simulink library "ctc"  (Simulink 8.1)
settings: Solver=ode1  StartTime=0.0  StopTime=Inf  FixedStep=0.001  RelTol=1e-3
PostLoadFcn:
  | , if any(exist('dsrtsu_mdlpostloadfcn', 'file') == [2, 3, 6]), try dsrtsu_mdlpostloadfcn('Execute', bdroot); catch fprintf('Error in PostLoadFcn (dsrtsu_mdlpostloadfcn) for model "%s":\n %s\n', bdroot, lasterr); end, end,
undefined symbols (not defined in the file or in its folder): ENUM_ACCSTATE_STANDSTILL, KACC_BackToTqMinDecel_mps2, ZERO_FLOAT
libraries: ctp x1, trs x1, ptc x1, ltt x1, tpl x1, tru x1, trl x1
settings Model: DSRTSU_INTERNAL_RTI_VER=450  DSRTSU_INTERNAL_RTI_TYPE=rti1401  RTICANMMDATA=struct('GeneralSetupData',struct('modelroot','D:\ELN150201_TAIWAN\trunk\AdasDragon\software\sw_development\arch\app\acc','generalsettings',struct('filesettings',struct('destfolder',struct('Name','RTICANMM_FILES','Check',1),'buildfolder',struct('Name','.','Check',1),'AbsDestfolder',struct('Name','D:\ELN150201_TAIWAN\trunk\AdasDragon\software\sw_development\arch\app\acc\RTICANMM_FILES'),'AbsBuildfolder',struct('Name','D:\ELN150201_TAIWAN\trunk\AdasDragon\software\sw_development\arch\app\acc'))),'options',struct('addpaths',1,'rmpaths',1,'addtrcexclusion',logical(1),'cannavigator',struct('checkmonitoring',0),'show_usrtrc',0,'use_usrtrc',0),'advanced',struct('options',[1 1 1 1 1 1 1 1 1 1 1 1 1 1 1 1 1 1 1 1 1 1 1 1 1 1 1 1 1 1 1 1 1 1 1 1 1 1 1 1 1 1 1 1 1 1 1 1 1 1 1 1 1 1 1 1 1 1 1 1 1 1 1 1 1 1 1 1 1 1 1 1 1 1 1 1 1 1 1 1 1 1 1 1 1 1 1 1 1 1 1 1 1 1 1 1 1 1 1 1]),'MPSetup',{{}},'modelname','ctc','block','ctc'))  DSRTSU_INTERNAL_RTIFPGA=40  Creator=tescamilla  LastModifiedBy=AT015555

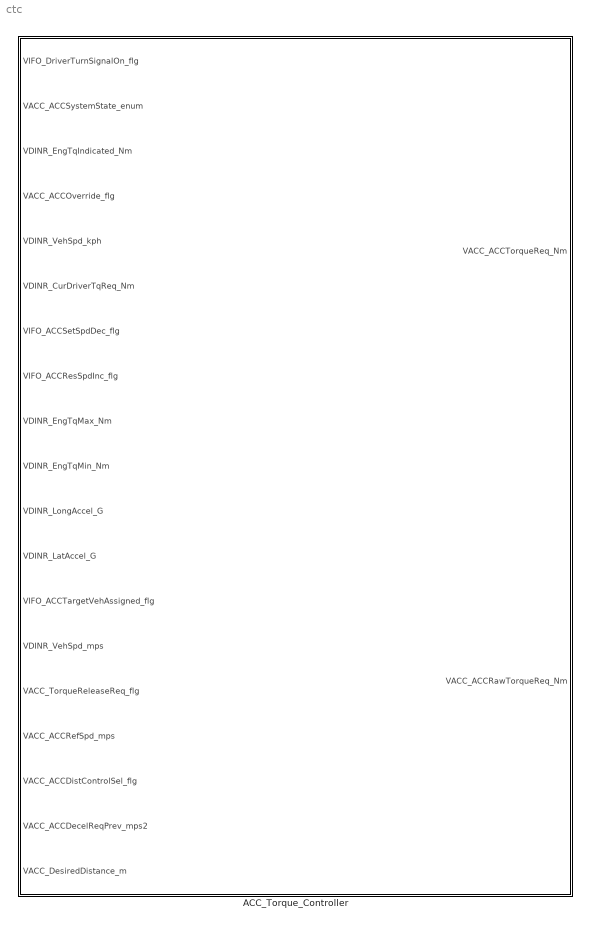
== system ctc ==
  ACC_Torque_Controller : Subsystem

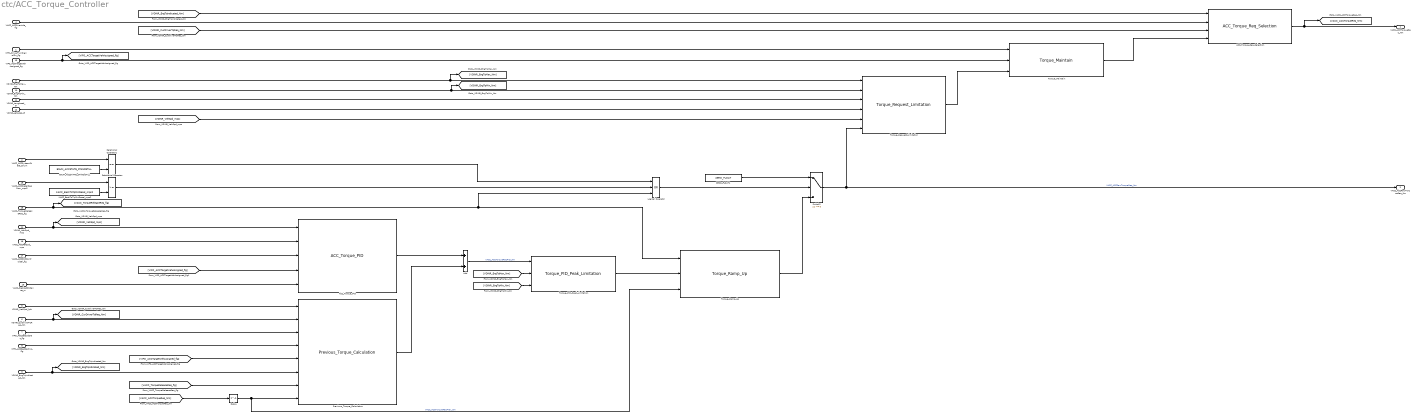
== system ctc/ACC_Torque_Controller ==
  VIFO_DriverTurnSignalOn_flg : Inport
  VACC_ACCSystemState_enum : Inport  Port=2
  VDINR_EngTqIndicated_Nm : Inport  Port=3
  VACC_ACCOverride_flg : Inport  Port=4
  VDINR_VehSpd_kph : Inport  Port=5
  VDINR_CurDriverTqReq_Nm : Inport  Port=6
  VIFO_ACCSetSpdDec_flg : Inport  Port=7
  VIFO_ACCResSpdInc_flg : Inport  Port=8
  VDINR_EngTqMax_Nm : Inport  Port=9
  VDINR_EngTqMin_Nm : Inport  Port=10
  VDINR_LongAccel_G : Inport  Port=11
  VDINR_LatAccel_G : Inport  Port=12
  VIFO_ACCTargetVehAssigned_flg : Inport  Port=13
  VDINR_VehSpd_mps : Inport  Port=14
  VACC_TorqueReleaseReq_flg : Inport  Port=15
  VACC_ACCRefSpd_mps : Inport  Port=16
  VACC_ACCDistControlSel_flg : Inport  Port=17
  VACC_ACCDecelReqPrev_mps2 : Inport  Port=18
  VACC_DesiredDistance_m : Inport  Port=19
  ACC_Torque_PID : ctp/ACC_Torque_PID
  ACC_Torque_Req_Selection : trs/ACC_Torque_Req_Selection
  Add : Sum
  Delay : Delay  DelayLength=1  InitialCondition=0
  ENUM_ACCSTATE_STANDSTILL : Constant  Value=ENUM_ACCSTATE_STANDSTILL
  KACC_BackToTqMinDecel_mps2 : Constant  Value=KACC_BackToTqMinDecel_mps2
  Logical Operator : Logic  Operator=OR  Inputs=3  AllPortsSameDT=off  OutDataTypeStr=boolean
  Previous_Torque_Calculation : ptc/Previous_Torque_Calculation
  Relational Operator : RelationalOperator  OutDataTypeStr=boolean
  Relational Operator1 : RelationalOperator  Operator===  OutDataTypeStr=boolean
  Switch2 : Switch  Criteria=u2 ~= 0
  Torque_Maintain : ltt/Torque_Maintain
  Torque_PID_Peak_Limitation : tpl/Torque_PID_Peak_Limitation
  Torque_Ramp_Up : tru/Torque_Ramp_Up
  Torque_Request_Limitation : trl/Torque_Request_Limitation
  ZERO_FLOAT1 : Constant  Value=ZERO_FLOAT
  VACC_ACCTorqueReq_Nm : Outport
  VACC_ACCRawTorqueReq_Nm : Outport  Port=2
  wires:
  VACC_ACCOverride_flg/1 -> ACC_Torque_Req_Selection/2
  [VDINR_CurDriverTqReq_Nm] -> ACC_Torque_Req_Selection/3
  [VDINR_VehSpd_mps] -> Torque_Request_Limitation/5
  VDINR_LatAccel_G/1 -> Torque_Request_Limitation/4
  VDINR_LongAccel_G/1 -> Torque_Request_Limitation/3
  VDINR_EngTqMax_Nm/1 -> [VDINR_EngTqMax_Nm], Torque_Request_Limitation/1
  VDINR_EngTqMin_Nm/1 -> [VDINR_EngTqMin_Nm], Torque_Request_Limitation/2
  Previous_Torque_Calculation/1 -> Add/2
  ACC_Torque_PID/1 -> Add/1
  Delay/1 -> Torque_Ramp_Up/3, Previous_Torque_Calculation/8  "VACC_ACCTorqueReqPrev_Nm"
  VIFO_ACCResSpdInc_flg/1 -> Previous_Torque_Calculation/4
  VIFO_ACCSetSpdDec_flg/1 -> Previous_Torque_Calculation/3
  VDINR_CurDriverTqReq_Nm/1 -> [VDINR_CurDriverTqReq_Nm], Previous_Torque_Calculation/2
  VDINR_VehSpd_kph/1 -> Previous_Torque_Calculation/1
  VDINR_VehSpd_mps/1 -> ACC_Torque_PID/1, [VDINR_VehSpd_mps]
  VACC_ACCRefSpd_mps/1 -> ACC_Torque_PID/2
  VACC_TorqueReleaseReq_flg/1 -> [VACC_TorqueReleaseReq_flg], Logical Operator/3, Torque_Ramp_Up/1
  ZERO_FLOAT1/1 -> Switch2/1
  Switch2/1 -> VACC_ACCRawTorqueReq_Nm/1, Torque_Request_Limitation/6  "VACC_ACCRawTorqueReq_Nm"
  Torque_Ramp_Up/1 -> Switch2/3
  VDINR_EngTqIndicated_Nm/1 -> [VDINR_EngTqIndicated_Nm], Previous_Torque_Calculation/6
  VACC_ACCDistControlSel_flg/1 -> ACC_Torque_PID/3
  [VACC_TorqueReleaseReq_flg] -> Previous_Torque_Calculation/7
  KACC_BackToTqMinDecel_mps2/1 -> Relational Operator/2
  VACC_ACCDecelReqPrev_mps2/1 -> Relational Operator/1
  Relational Operator/1 -> Logical Operator/2
  Logical Operator/1 -> Switch2/2
  VACC_ACCSystemState_enum/1 -> Relational Operator1/1
  ENUM_ACCSTATE_STANDSTILL/1 -> Relational Operator1/2
  Relational Operator1/1 -> Logical Operator/1
  Add/1 -> Torque_PID_Peak_Limitation/1  "VACC_ACCTorqueReqPID_Nm"
  [VDINR_EngTqMax_Nm] -> Torque_PID_Peak_Limitation/2
  [VDINR_EngTqMin_Nm] -> Torque_PID_Peak_Limitation/3
  Torque_PID_Peak_Limitation/1 -> Torque_Ramp_Up/2
  ACC_Torque_Req_Selection/1 -> [VACC_ACCTorqueReq_Nm], VACC_ACCTorqueReq_Nm/1
  VIFO_ACCTargetVehAssigned_flg/1 -> [VIFO_ACCTargetVehAssigned_flg], Torque_Maintain/2
  [VIFO_ACCTargetVehAssigned_flg] -> Previous_Torque_Calculation/5
  Torque_Request_Limitation/1 -> Torque_Maintain/3
  Torque_Maintain/1 -> ACC_Torque_Req_Selection/4
  [VDINR_EngTqIndicated_Nm] -> ACC_Torque_Req_Selection/1
  [VIFO_ACCTargetVehAssigned_flg] -> ACC_Torque_PID/4
  VACC_DesiredDistance_m/1 -> ACC_Torque_PID/5
  [VACC_ACCTorqueReq_Nm] -> Delay/1
  VIFO_DriverTurnSignalOn_flg/1 -> Torque_Maintain/1
